simulink model "automata_learning"  (R2021b)
settings: Solver=VariableStepAuto  StartTime=0.0  StopTime=10.0  RelTol=1e-3
settings Model: Creator=Falk  LastModifiedBy=Falk

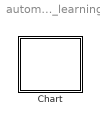
== system automata_learning ==
  Chart : Stateflow chart  TreatAsAtomicUnit=on

== stateflow chart automata_learning/Chart ==
